simulink model "W08_0_offline"  (R2024b)
settings: Solver=ode4  StartTime=0.0  StopTime=T_end  FixedStep=Ts_ctrl  RelTol=1e-3
values from neighbouring files (symbols this model uses):
  A_Fw = 1.5    [W08_setup.m]
  A_Lw = 3.0    (= 3)    [W08_setup.m]
  alloc_mode = 2    [W08_setup.m]
  animate = 1    [W08_setup.m]
  c_n = 0.12    [W08_setup.m]
  c_x = 0.70    (= 0.7)    [W08_setup.m]
  c_y = 0.85    [W08_setup.m]
  del_max = deg2rad(45)    [W08_setup.m]
  del_rate = deg2rad(30)    [W08_setup.m]
  dp_E0 = 0    [W08_setup.m]
  dp_mode = 1    [W08_setup.m]
  dp_N0 = 0    [W08_setup.m]
  dp_PSI0 = deg2rad(0)    [W08_setup.m]
  dp_ref_on = 1    [W08_setup.m]
  dp_step = [  0    0     0    0 ... (first row only)    [W08_setup.m]
  dp_vmax = [0.5; 0.5; deg2rad(8)]    [W08_setup.m]
  F_max = 500    [W08_setup.m]
  filt_on = 1    [W08_setup.m]
  i_max = [ 200; 200; 400 ]    [W08_setup.m]
  k_wave = 900    [W08_setup.m]
  Kd_dp = diag([  110,   110,   200 ])    [W08_setup.m]
  Ki_dp = diag([    5,     5,    16 ])    [W08_setup.m]
  Kp_dp = diag([   50,    50,   160 ])    [W08_setup.m]
  L_oa = 4.9    [W08_setup.m]
  lw_arm = 1.2    [W08_setup.m]
  plant_par = [m_usv; Izz; Xu; Xuu; Yv; Yvv; Nr; Nrr]    [W08_setup.m]
  rho_air = 1.225    [W08_setup.m]
  T_e = [     1,      0,      1,      0 ... (first row only)    [W08_setup.m]
  T_pinv = pinv(T_e)    [W08_setup.m]    (also in W08_sway_demo.m = evalin('base','T_pinv'); W10_sway_demo.m = evalin('base','T_pinv'))
  tau_del = 0.20    (= 0.2)    [W08_setup.m]
  tau_n = 0.30    (= 0.3)    [W08_setup.m]
  tau_ref = 6    [W08_setup.m]
  Ts_ctrl = 0.05    [W08_setup.m]
  w_filt = 1.20    (= 1.2)    [W08_setup.m]
  wave_dir = deg2rad(45)    [W08_setup.m]
  wave_on = 1    [W08_setup.m]
  wave_par = [w_i, A_i, phi_i]    [W08_setup.m]
  wind_dir = deg2rad(45)    [W08_setup.m]
  wind_on = 1    [W08_setup.m]
  wind_speed = 6.0    (= 6)    [W08_setup.m]
  x0 = [0; 0; 0; 0; 0; 0]    [W08_setup.m]    (also in W08_vrx_run.m = x0old;   x0(6) = psi0;   assignin('base','x0', x0))
settings Model: Creator=admin  LastModifiedBy=admin

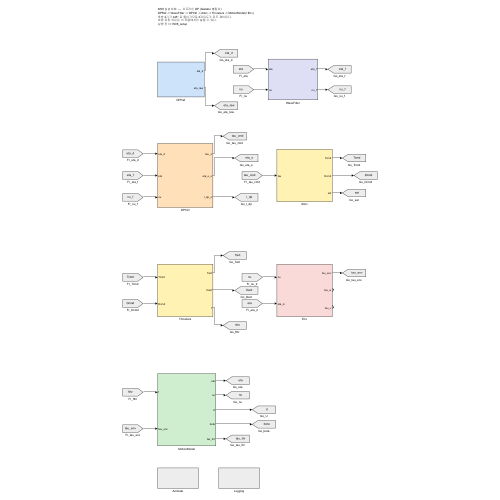
[thumbnail: Simulink's stored preview of the top-level diagram]
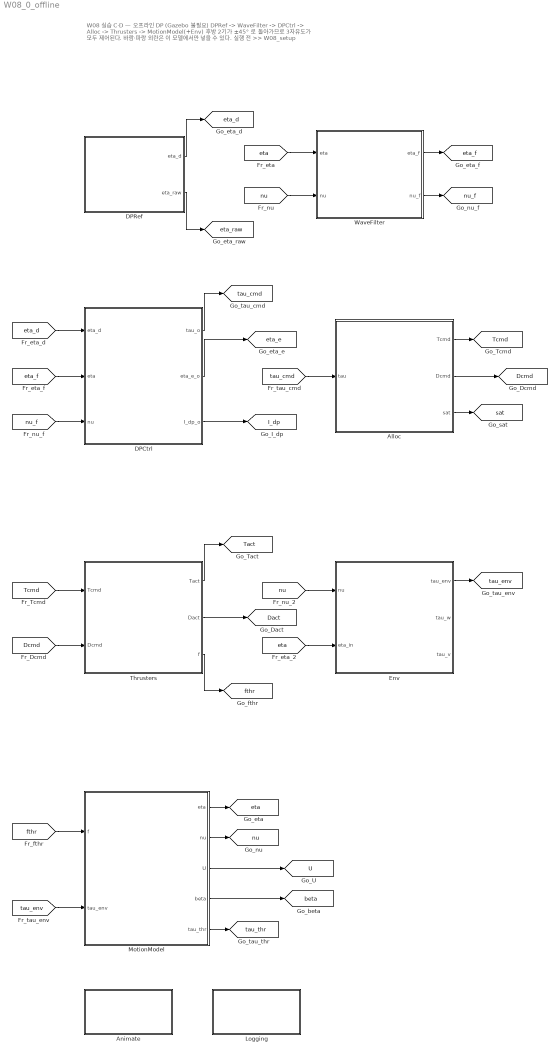
== system W08_0_offline ==
  note: W08 실습 C·D  —  오프라인 DP (Gazebo 불필요)
      | DPRef -> WaveFilter -> DPCtrl -> Alloc -> Thrusters -> MotionModel(+Env)
      | 후방 2기가 ±45° 로 돌아가므로 3자유도가 모두 제어된다.
      | 바람·파랑 외란은 이 모델에서만 넣을 수 있다.
      | 실행 전 >> W08_setup
  Alloc : Subsystem
  Animate : Subsystem
  DPCtrl : Subsystem
  DPRef : Subsystem
  Env : Subsystem
  Logging : Subsystem
  MotionModel : Subsystem
  Thrusters : Subsystem
  WaveFilter : Subsystem
  tag scope: Dact=global, Dcmd=global, I_dp=global, Tact=global, Tcmd=global, U=global, beta=global, eta=global, eta_d=global, eta_e=global, eta_f=global, eta_raw=global, fthr=global, nu=global, nu_f=global, sat=global, tau_cmd=global, tau_env=global, tau_thr=global
  wires:
  [tau_env] -> MotionModel/2(tau_env)
  [fthr] -> MotionModel/1(f)
  [eta] -> Env/2(eta_in)
  [nu] -> Env/1(nu)
  [Dcmd] -> Thrusters/2(Dcmd)
  [Tcmd] -> Thrusters/1(Tcmd)
  [tau_cmd] -> Alloc/1(tau)
  [nu_f] -> DPCtrl/3(nu)
  [eta_f] -> DPCtrl/2(eta)
  [eta_d] -> DPCtrl/1(eta_d)
  [nu] -> WaveFilter/2(nu)
  [eta] -> WaveFilter/1(eta)
  Thrusters/2(Dact) -> [Dact]
  Alloc/2(Dcmd) -> [Dcmd]
  DPCtrl/3(I_dp_o) -> [I_dp]
  Thrusters/1(Tact) -> [Tact]
  Alloc/1(Tcmd) -> [Tcmd]
  MotionModel/3(U) -> [U]
  MotionModel/4(beta) -> [beta]
  MotionModel/1(eta) -> [eta]
  DPRef/1(eta_d) -> [eta_d]
  DPCtrl/2(eta_e_o) -> [eta_e]
  WaveFilter/1(eta_f) -> [eta_f]
  DPRef/2(eta_raw) -> [eta_raw]
  Thrusters/3(f) -> [fthr]
  MotionModel/2(nu) -> [nu]
  WaveFilter/2(nu_f) -> [nu_f]
  Alloc/3(sat) -> [sat]
  DPCtrl/1(tau_o) -> [tau_cmd]
  Env/1(tau_env) -> [tau_env]
  MotionModel/5(tau_thr) -> [tau_thr]

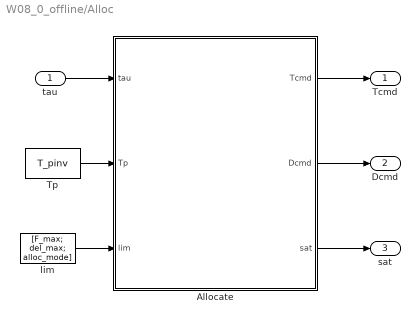
== system W08_0_offline/Alloc ==
  tau : Inport
  Allocate : MATLAB Function  TreatAsAtomicUnit=on
  Tp : Constant  Value=T_pinv
  lim : Constant  Value=[F_max; del_max; alloc_mode]
  Tcmd : Outport
  Dcmd : Outport  Port=2
  sat : Outport  Port=3
  wires:
  lim/1 -> Allocate/3(lim)
  tau/1 -> Allocate/1(tau)
  Allocate/2(Dcmd) -> Dcmd/1
  Tp/1 -> Allocate/2(Tp)
  Allocate/1(Tcmd) -> Tcmd/1
  Allocate/3(sat) -> sat/1

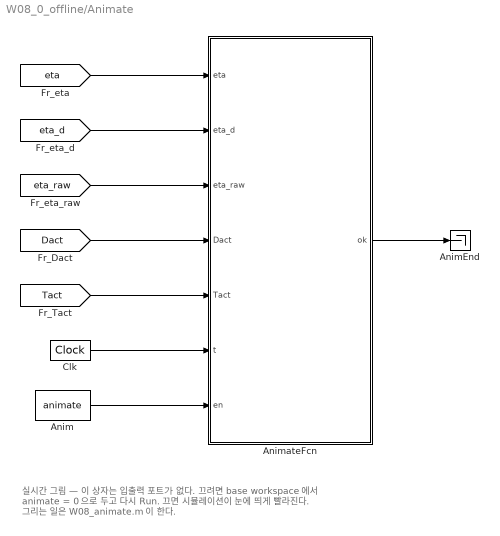
== system W08_0_offline/Animate ==
  note: 실시간 그림 — 이 상자는 입출력 포트가 없다.
      | 끄려면 base workspace 에서  animate = 0  으로 두고 다시 Run.
      | 끄면 시뮬레이션이 눈에 띄게 빨라진다.
      | 그리는 일은 W08_animate.m 이 한다.
  Anim : Constant  Value=animate
  AnimEnd : Terminator
  AnimateFcn : MATLAB Function  TreatAsAtomicUnit=on
  Clk : DigitalClock  SampleTime=Ts_ctrl
  wires:
  [eta] -> AnimateFcn/1(eta)
  [eta_d] -> AnimateFcn/2(eta_d)
  [eta_raw] -> AnimateFcn/3(eta_raw)
  [Dact] -> AnimateFcn/4(Dact)
  [Tact] -> AnimateFcn/5(Tact)
  Clk/1 -> AnimateFcn/6(t)
  Anim/1 -> AnimateFcn/7(en)
  AnimateFcn/1(ok) -> AnimEnd/1

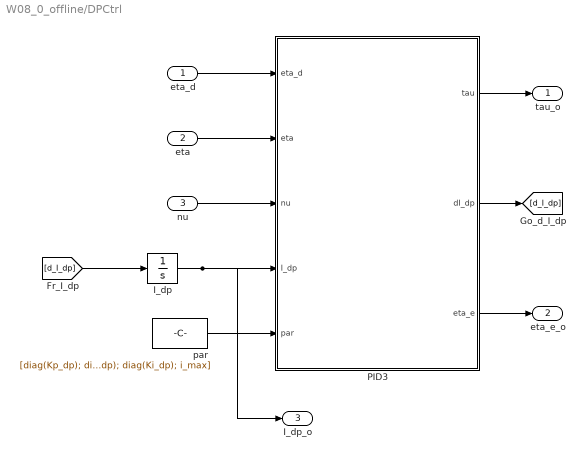
== system W08_0_offline/DPCtrl ==
  eta_d : Inport
  eta : Inport  Port=2
  nu : Inport  Port=3
  I_dp : Integrator  InitialCondition=[0;0;0]
  PID3 : MATLAB Function  TreatAsAtomicUnit=on
  par : Constant  Value=[diag(Kp_dp); diag(Kd_dp); diag(Ki_dp); i_max]
  tau_o : Outport
  eta_e_o : Outport  Port=2
  I_dp_o : Outport  Port=3
  wires:
  [d_I_dp] -> I_dp/1
  I_dp/1 -> PID3/4(I_dp), I_dp_o/1
  eta_d/1 -> PID3/1(eta_d)
  PID3/1(tau) -> tau_o/1
  eta/1 -> PID3/2(eta)
  par/1 -> PID3/5(par)
  nu/1 -> PID3/3(nu)
  PID3/2(dI_dp) -> [d_I_dp]
  PID3/3(eta_e) -> eta_e_o/1

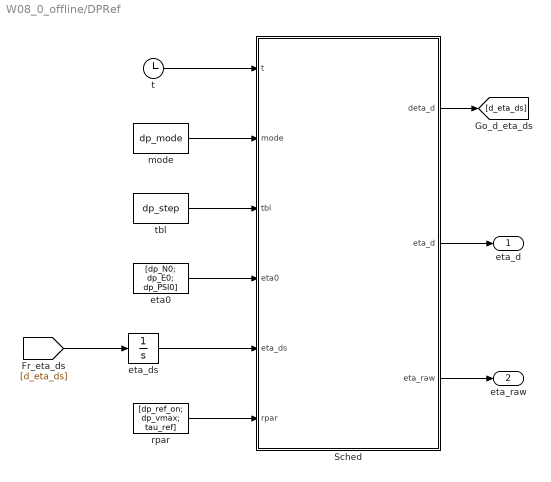
== system W08_0_offline/DPRef ==
  Sched : MATLAB Function  TreatAsAtomicUnit=on
  eta0 : Constant  Value=[dp_N0; dp_E0; dp_PSI0]
  eta_ds : Integrator  InitialCondition=[dp_N0; dp_E0; dp_PSI0]
  mode : Constant  Value=dp_mode
  rpar : Constant  Value=[dp_ref_on; dp_vmax; tau_ref]
  t : Clock
  tbl : Constant  Value=dp_step
  eta_d : Outport
  eta_raw : Outport  Port=2
  wires:
  [d_eta_ds] -> eta_ds/1
  Sched/1(deta_d) -> [d_eta_ds]
  t/1 -> Sched/1(t)
  mode/1 -> Sched/2(mode)
  eta_ds/1 -> Sched/5(eta_ds)
  tbl/1 -> Sched/3(tbl)
  eta0/1 -> Sched/4(eta0)
  rpar/1 -> Sched/6(rpar)
  Sched/2(eta_d) -> eta_d/1
  Sched/3(eta_raw) -> eta_raw/1

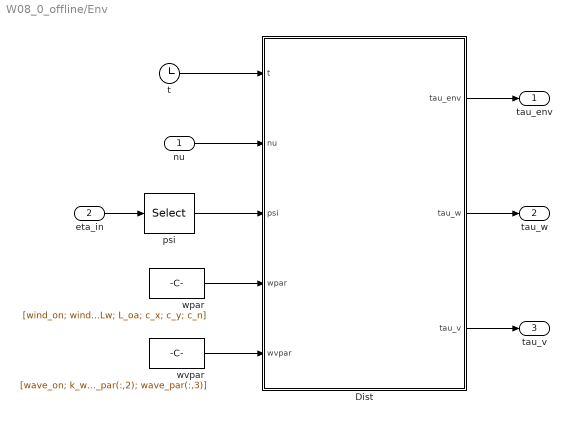
== system W08_0_offline/Env ==
  nu : Inport
  eta_in : Inport  Port=2
  Dist : MATLAB Function  TreatAsAtomicUnit=on
  psi : Selector  InputPortWidth=3  IndexOptions=Index vector (dialog)  Indices=3  OutputSizes=1
  t : Clock
  wpar : Constant  Value=[wind_on; wind_speed; wind_dir; rho_air; A_Fw; A_Lw; L_oa; c_x; c_y; c_n]
  wvpar : Constant  Value=[wave_on; k_wave; wave_dir; lw_arm; wave_par(:,1); wave_par(:,2); wave_par(:,3)]
  tau_env : Outport
  tau_w : Outport  Port=2
  tau_v : Outport  Port=3
  wires:
  eta_in/1 -> psi/1
  Dist/1(tau_env) -> tau_env/1
  t/1 -> Dist/1(t)
  nu/1 -> Dist/2(nu)
  psi/1 -> Dist/3(psi)
  wvpar/1 -> Dist/5(wvpar)
  Dist/3(tau_v) -> tau_v/1
  wpar/1 -> Dist/4(wpar)
  Dist/2(tau_w) -> tau_w/1

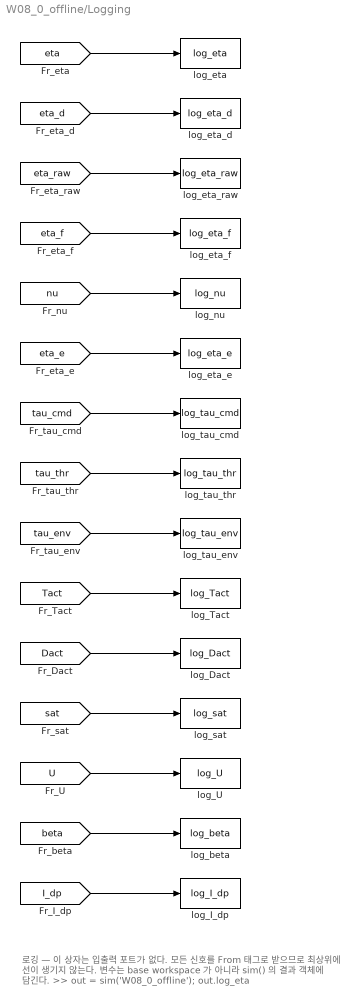
== system W08_0_offline/Logging ==
  note: 로깅 — 이 상자는 입출력 포트가 없다.
      | 모든 신호를 From 태그로 받으므로 최상위에 선이 생기지 않는다.
      | 변수는 base workspace 가 아니라 sim() 의 결과 객체에 담긴다.
      |   >> out = sim('W08_0_offline');  out.log_eta
  log_Dact : ToWorkspace  VariableName=log_Dact  SaveFormat=Timeseries  SampleTime=Ts_ctrl
  log_I_dp : ToWorkspace  VariableName=log_I_dp  SaveFormat=Timeseries  SampleTime=Ts_ctrl
  log_Tact : ToWorkspace  VariableName=log_Tact  SaveFormat=Timeseries  SampleTime=Ts_ctrl
  log_U : ToWorkspace  VariableName=log_U  SaveFormat=Timeseries  SampleTime=Ts_ctrl
  log_beta : ToWorkspace  VariableName=log_beta  SaveFormat=Timeseries  SampleTime=Ts_ctrl
  log_eta : ToWorkspace  VariableName=log_eta  SaveFormat=Timeseries  SampleTime=Ts_ctrl
  log_eta_d : ToWorkspace  VariableName=log_eta_d  SaveFormat=Timeseries  SampleTime=Ts_ctrl
  log_eta_e : ToWorkspace  VariableName=log_eta_e  SaveFormat=Timeseries  SampleTime=Ts_ctrl
  log_eta_f : ToWorkspace  VariableName=log_eta_f  SaveFormat=Timeseries  SampleTime=Ts_ctrl
  log_eta_raw : ToWorkspace  VariableName=log_eta_raw  SaveFormat=Timeseries  SampleTime=Ts_ctrl
  log_nu : ToWorkspace  VariableName=log_nu  SaveFormat=Timeseries  SampleTime=Ts_ctrl
  log_sat : ToWorkspace  VariableName=log_sat  SaveFormat=Timeseries  SampleTime=Ts_ctrl
  log_tau_cmd : ToWorkspace  VariableName=log_tau_cmd  SaveFormat=Timeseries  SampleTime=Ts_ctrl
  log_tau_env : ToWorkspace  VariableName=log_tau_env  SaveFormat=Timeseries  SampleTime=Ts_ctrl
  log_tau_thr : ToWorkspace  VariableName=log_tau_thr  SaveFormat=Timeseries  SampleTime=Ts_ctrl
  wires:
  [eta] -> log_eta/1
  [eta_d] -> log_eta_d/1
  [eta_raw] -> log_eta_raw/1
  [eta_f] -> log_eta_f/1
  [nu] -> log_nu/1
  [eta_e] -> log_eta_e/1
  [tau_cmd] -> log_tau_cmd/1
  [tau_thr] -> log_tau_thr/1
  [tau_env] -> log_tau_env/1
  [Tact] -> log_Tact/1
  [Dact] -> log_Dact/1
  [sat] -> log_sat/1
  [U] -> log_U/1
  [beta] -> log_beta/1
  [I_dp] -> log_I_dp/1

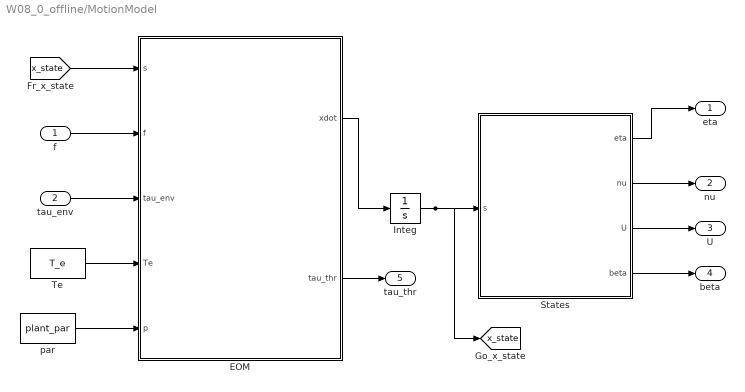
== system W08_0_offline/MotionModel ==
  f : Inport
  tau_env : Inport  Port=2
  EOM : MATLAB Function  TreatAsAtomicUnit=on
  Integ : Integrator  InitialCondition=x0
  States : MATLAB Function  TreatAsAtomicUnit=on
  Te : Constant  Value=T_e
  par : Constant  Value=plant_par
  eta : Outport
  nu : Outport  Port=2
  U : Outport  Port=3
  beta : Outport  Port=4
  tau_thr : Outport  Port=5
  tag scope: x_state=global
  wires:
  f/1 -> EOM/2(f)
  [x_state] -> EOM/1(s)
  EOM/1(xdot) -> Integ/1
  tau_env/1 -> EOM/3(tau_env)
  par/1 -> EOM/5(p)
  Te/1 -> EOM/4(Te)
  Integ/1 -> States/1(s), [x_state]
  EOM/2(tau_thr) -> tau_thr/1
  States/1(eta) -> eta/1
  States/2(nu) -> nu/1
  States/3(U) -> U/1
  States/4(beta) -> beta/1

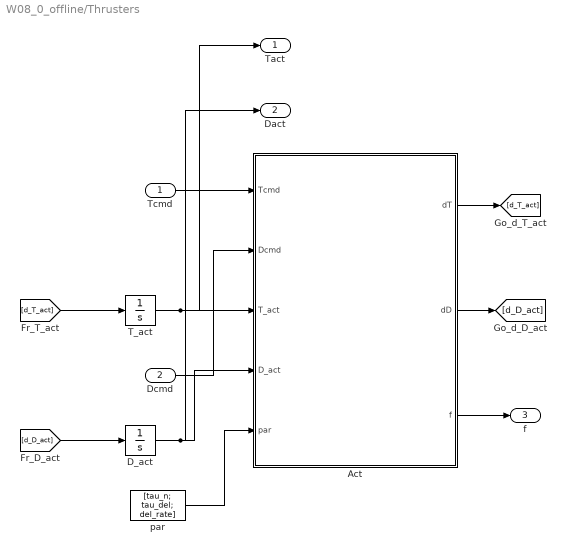
== system W08_0_offline/Thrusters ==
  Tcmd : Inport
  Dcmd : Inport  Port=2
  Act : MATLAB Function  TreatAsAtomicUnit=on
  D_act : Integrator  InitialCondition=[0;0]
  T_act : Integrator  InitialCondition=[0;0]
  par : Constant  Value=[tau_n; tau_del; del_rate]
  Tact : Outport
  Dact : Outport  Port=2
  f : Outport  Port=3
  wires:
  [d_T_act] -> T_act/1
  Tcmd/1 -> Act/1(Tcmd)
  [d_D_act] -> D_act/1
  T_act/1 -> Tact/1, Act/3(T_act)
  Act/1(dT) -> [d_T_act]
  par/1 -> Act/5(par)
  Dcmd/1 -> Act/2(Dcmd)
  D_act/1 -> Dact/1, Act/4(D_act)
  Act/2(dD) -> [d_D_act]
  Act/3(f) -> f/1

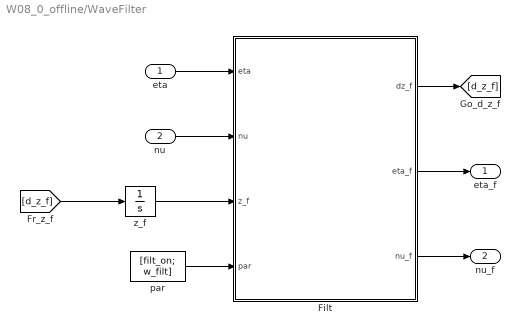
== system W08_0_offline/WaveFilter ==
  eta : Inport
  nu : Inport  Port=2
  Filt : MATLAB Function  TreatAsAtomicUnit=on
  par : Constant  Value=[filt_on; w_filt]
  z_f : Integrator  InitialCondition=[0;0;0;0;0;0]
  eta_f : Outport
  nu_f : Outport  Port=2
  wires:
  [d_z_f] -> z_f/1
  Filt/2(eta_f) -> eta_f/1
  par/1 -> Filt/4(par)
  z_f/1 -> Filt/3(z_f)
  eta/1 -> Filt/1(eta)
  nu/1 -> Filt/2(nu)
  Filt/1(dz_f) -> [d_z_f]
  Filt/3(nu_f) -> nu_f/1

== matlab function W08_0_offline/MotionModel/States ==
  data: s input; eta output; nu output; U output; beta output
function [eta, nu, U, beta] = States(s)
%#codegen
nu   = s(1:3);
eta  = s(4:6);
U    = sqrt(s(1)*s(1) + s(2)*s(2));
beta = atan2(s(2), s(1));

== matlab function W08_0_offline/Animate/AnimateFcn ==
  data: eta input; ok output; eta_d input; eta_raw input; Dact input; Tact input; t input; en input
function ok = AnimateFcn(eta, eta_d, eta_raw, Dact, Tact, t, en)
%#codegen
% Live plot while the model runs. A MATLAB Function block cannot
% plot, so the drawing function is declared extrinsic: Simulink
% calls plain MATLAB instead of generating code for it.
coder.extrinsic('W08_animate');
ok = 1;
if en > 0.5
    W08_animate(eta, eta_d, eta_raw, Dact, Tact, t);
end

== matlab function W08_0_offline/WaveFilter/Filt ==
  data: eta input; dz_f output; nu input; z_f input; par input; eta_f output; nu_f output
function [dz_f, eta_f, nu_f] = Filt(eta, nu, z_f, par)
%#codegen
% Wave filtering for dynamic positioning.
%
% First order wave loads make the vessel oscillate at the wave
% frequency. That motion cannot be counteracted — trying to do so
% only wears out the thrusters. A DP system therefore feeds the
% controller with the LOW FREQUENCY part of the motion only.
% Fossen (2011) 11.4.1 uses a passive observer; here a first order
% low pass with a cut-off well below the wave frequency is enough to
% show the effect.
%
% CONTINUOUS TIME:   dz_f/dt = wf * (z - z_f)
% An Integrator holds z_f, so the cut-off wf is the only number here.
%
% par = [on; wf]

on = par(1); wf = par(2);
z  = [eta; nu];
dz_f = zeros(6,1);
if on < 0.5
    eta_f = eta;  nu_f = nu;
    return
end
d = z - z_f;
% heading must be filtered on the difference, not the raw angle
d(3) = atan2(sin(d(3)), cos(d(3)));
dz_f = wf * d;
eta_f = z_f(1:3);
nu_f  = z_f(4:6);

== matlab function W08_0_offline/DPRef/Sched ==
  data: t input; deta_d output; mode input; tbl input; eta0 input; eta_ds input; rpar input; eta_d output; eta_raw output
function [deta_d, eta_d, eta_raw] = Sched(t, mode, tbl, eta0, eta_ds, rpar)
%#codegen
% DP setpoint scheduler and REFERENCE MODEL.
%
%   mode 0 : hold the initial setpoint
%   mode 1 : step through the table  [t  N  E  psi_deg]
%
% A raw step demand is never given to a DP controller. The vessel
% cannot move at any speed, so a step makes the controller ask for a
% force the thrusters cannot deliver, and the loop saturates.
% A reference model turns the step into a feasible trajectory. Here a
% saturated proportional law is used:
%     v = (eta_raw - eta_d)/tau_ref,   |v| <= v_max
% Far from the target the setpoint moves at the constant speed v_max;
% close to it the approach becomes exponential with time constant
% tau_ref, so there is no corner at arrival.
% Fossen (2011) calls this the reference model; every DP system has
% one.
%
% CONTINUOUS TIME. The function returns the RATE of the setpoint and
% an Integrator holds the state, so the law above is written exactly
% as it stands - no Ts anywhere.
%
% rpar = [on; vx; vy; vPsi; tau_ref]

eta_raw = eta0;
if mode > 0.5
    n = size(tbl,1);
    for i = 1:n
        if t >= tbl(i,1)
            eta_raw = [tbl(i,2); tbl(i,3); tbl(i,4)*pi/180];
        end
    end
end

deta_d = zeros(3,1);
if rpar(1) < 0.5
    eta_d = eta_raw;        % reference model off: the step goes straight through
    return
end

vmax = rpar(2:4);  tr = rpar(5);
for i = 1:3
    d = eta_raw(i) - eta_ds(i);
    if i == 3, d = atan2(sin(d), cos(d)); end
    v = d/tr;
    if v >  vmax(i), v =  vmax(i); end
    if v < -vmax(i), v = -vmax(i); end
    deta_d(i) = v;
end
eta_d = eta_ds;

== matlab function W08_0_offline/DPCtrl/PID3 ==
  data: eta_d input; tau output; eta input; nu input; I_dp input; par input; dI_dp output; eta_e output
function [tau, dI_dp, eta_e] = PID3(eta_d, eta, nu, I_dp, par)
%#codegen
% 3-DOF dynamic positioning controller (Fossen 2011, 12.2.10).
%
%   eta   = [N; E; psi]      position and heading in NED
%   nu    = [u; v; r]        velocity in BODY
%   tau   = -J(psi)' * (Kp*eta_e + Ki*I) - Kd*nu
%
% The transpose of the rotation matrix turns a NED position error into
% a BODY force. Damping is taken on BODY velocity directly, so no
% derivative of the error is needed (same idea as the P-D heading
% controller of week 7).
%
% CONTINUOUS TIME. The function returns dI/dt = e and an Integrator
% holds I, so the integral term is a true 1/s - there is no Ts here.
%
% par = [Kp(1:3); Kd(1:3); Ki(1:3); imax(1:3)]

Kp = par(1:3);  Kd = par(4:6);  Ki = par(7:9);  im = par(10:12);

e = eta - eta_d;
e(3) = atan2(sin(e(3)), cos(e(3)));      % smallest signed angle

psi = eta(3);
J = [ cos(psi), -sin(psi), 0;
      sin(psi),  cos(psi), 0;
             0,         0, 1];

% CLAMPING anti-windup: at the limit, and still being pushed further
% out, the integral simply stops. Same rule the PI blocks of weeks
% 4-7 use, written out because the law here is 3-DOF.
dI_dp = e;
for i = 1:3
    lim = im(i)/max(Ki(i), 1e-9);
    if (I_dp(i) >=  lim && e(i) > 0) || (I_dp(i) <= -lim && e(i) < 0)
        dI_dp(i) = 0;
    end
end

tau = -J' * ( Kp.*e + Ki.*I_dp ) - Kd.*nu;
eta_e = e;

== matlab function W08_0_offline/Alloc/Allocate ==
  data: tau input; Tcmd output; Tp input; lim input; Dcmd output; sat output
function [Tcmd, Dcmd, sat] = Allocate(tau, Tp, lim)
%#codegen
% Thrust allocation for two azimuth (rotatable) thrusters.
% Fossen (2011) 12.3.4 — constrained control allocation for azimuth
% thrusters, solved with the EXTENDED THRUST VECTOR.
%
% Step 1  f = pinv(T_e) * tau       f = [FxL FyL FxR FyR]'
%         Because the thruster force is written in Cartesian components,
%         T_e is CONSTANT and its pseudo-inverse can be precomputed.
%         There is no singular configuration to worry about.
%
% Step 2  Cartesian -> polar   T = |f_i|,  delta = atan2(Fy, Fx)
%
% Step 3  map the demand into the mechanical sector |delta| <= 45 deg
%           |d| <=  45  : use as is
%           |d| >  135  : REVERSE thrust, d -> d -+ 180
%           otherwise   : dead zone, no thrust can be produced
%
% Step 4  saturate the magnitude at F_max
%
% lim = [F_max; delta_max; mode]
%   mode 1 : dead zone   — demands inside the forbidden sector are
%            dropped. Simple, but the realised tau is then wrong.
%   mode 2 : clamp       — the angle is pushed to the nearest sector
%            edge and the magnitude is scaled by cos of the angle
%            error, so the useful component is kept.

f = Tp * tau;
Fmax = lim(1);  dmax = lim(2);  mode = lim(3);

Tcmd = zeros(2,1);  Dcmd = zeros(2,1);  sat = 0;
for i = 1:2
    fx = f(2*i-1);  fy = f(2*i);
    Ti = sqrt(fx*fx + fy*fy);
    di = atan2(fy, fx);
    ad = abs(di);
    if ad <= dmax
        To = Ti;   Do = di;
    elseif ad >= pi - dmax
        To = -Ti;  Do = di - sign(di)*pi;    % reverse thrust
    elseif mode < 1.5
        To = 0;    Do = 0;                   % dead zone
        sat = sat + 1;
    else
        % clamp to the nearest edge of the reachable sector
        if ad <= pi/2
            Do = sign(di)*dmax;      To =  Ti*cos(ad - dmax);
        else
            Do = -sign(di)*dmax;        To = -Ti*cos(pi - dmax - ad);
            Do = atan2(sin(Do), cos(Do));
        end
        sat = sat + 1;
    end
    if To >  Fmax, To =  Fmax; sat = sat + 1; end
    if To < -Fmax, To = -Fmax; sat = sat + 1; end
    Tcmd(i) = To;  Dcmd(i) = Do;
end

== matlab function W08_0_offline/Thrusters/Act ==
  data: Tcmd input; dT output; Dcmd input; T_act input; D_act input; par input; dD output; f output
function [dT, dD, f] = Act(Tcmd, Dcmd, T_act, D_act, par)
%#codegen
% Actuator dynamics of an azimuth thruster.
%   thrust  : first order lag, time constant tau_n
%   azimuth : first order lag (tau_del) whose angular RATE is capped
%             at rate_max. A real pod cannot snap to a new angle.
%
% CONTINUOUS TIME. The function returns the two RATES and Integrators
% hold the states, so the rate cap is written on the rate itself -
% rad/s, not rad per sample.
%
%   dT/dt = (Tcmd - T)/tau_n
%   dD/dt = sat( ssa(Dcmd - D)/tau_del , +-rate_max )
%
% par = [tau_n; tau_del; rate_max]

tn = par(1); td = par(2); rmax = par(3);

dT = (Tcmd - T_act)/tn;

dD = zeros(2,1);
for i = 1:2
    dd = Dcmd(i) - D_act(i);
    dd = atan2(sin(dd), cos(dd));           % shortest way round
    rate = dd/td;                           % first order lag ...
    if rate >  rmax, rate =  rmax; end      % ... whose RATE is capped
    if rate < -rmax, rate = -rmax; end
    dD(i) = rate;
end

% back to Cartesian components in BODY
f = [ T_act(1)*cos(D_act(1));
      T_act(1)*sin(D_act(1));
      T_act(2)*cos(D_act(2));
      T_act(2)*sin(D_act(2)) ];

== matlab function W08_0_offline/Env/Dist ==
  data: t input; tau_env output; nu input; psi input; wpar input; wvpar input; tau_w output; tau_v output
function [tau_env, tau_w, tau_v] = Dist(t, nu, psi, wpar, wvpar)
%#codegen
% Environmental loads in BODY axes.
%
% WIND  — Jin et al. (2025) Eq. (11)-(19); Fossen (2011) 8.1
%   relative wind in BODY :
%     u_rw = u + Vw cos(beta_w - psi)   beta_w = direction wind COMES FROM
%     v_rw = v + Vw sin(beta_w - psi)   (Fossen uses going-to, hence minus)
%   q     = 0.5 rho_a Vrw^2
%   tau_w = q * [ CX*AFw ; CY*ALw ; CN*ALw*L ]
%   CX = -cx cos(g), CY = +cy sin(g), CN = cn sin(2g)   (Fossen 8.21)
%
% WAVE  — first order approximation. Component amplitudes come from a
%   Bretschneider spectrum (Jin et al. Eq. (21)-(25)); the force is
%   taken proportional to the surface elevation with a single gain.
%   This is an approximation, not a diffraction calculation.
%
% wpar  = [on; Vw; beta_w; rho_a; AFw; ALw; L; cx; cy; cn]
% wvpar = [on; k_wave; theta_m; arm; w1..wn; A1..An; p1..x_n]

u = nu(1); v = nu(2);
tau_w = zeros(3,1);
if wpar(1) > 0.5
    Vw = wpar(2); bw = wpar(3); rho = wpar(4);
    AF = wpar(5); AL = wpar(6); L = wpar(7);
    cx = wpar(8); cy = wpar(9); cn = wpar(10);
    urw = u + Vw*cos(bw - psi);
    vrw = v + Vw*sin(bw - psi);
    Vrw = sqrt(urw*urw + vrw*vrw);
    g   = -atan2(vrw, urw);
    q   = 0.5*rho*Vrw*Vrw;
    tau_w = q * [ -cx*cos(g)*AF;
                   cy*sin(g)*AL;
                   cn*sin(2*g)*AL*L ];
end

tau_v = zeros(3,1);
if wvpar(1) > 0.5
    kw = wvpar(2); th = wvpar(3); arm = wvpar(4);
    n  = (numel(wvpar) - 4)/3;
    zeta = 0;
    for i = 1:n
        wi = wvpar(4+i);
        Ai = wvpar(4+n+i);
        pi_i = wvpar(4+2*n+i);
        zeta = zeta + Ai*sin(wi*t + pi_i);
    end
    rel = th - psi;                          % wave direction in BODY
    Fw  = kw*zeta;
    tau_v = [ Fw*cos(rel); Fw*sin(rel); arm*Fw*sin(rel) ];
end

tau_env = tau_w + tau_v;

== matlab function W08_0_offline/MotionModel/EOM ==
  data: s input; xdot output; f input; tau_env input; Te input; p input; tau_thr output
function [xdot, tau_thr] = EOM(s, f, tau_env, Te, p)
%#codegen
% 3-DOF WAM-V equations of motion, NED — same coefficients as weeks
% 7 to 9 (taken from the Gazebo VRX plugins).
% The only change is the input: the thruster force now has a sway
% component, so all three degrees of freedom are actuated.
%   s = [u v r N E psi]'
%   p = [m Izz Xu Xuu Yv Yvv Nr Nrr]'

u = s(1); v = s(2); r = s(3); psi = s(6);
mm=p(1); Izz=p(2); Xu=p(3); Xuu=p(4); Yv=p(5); Yvv=p(6);
Nr=p(7); Nrr=p(8);

tau_thr = Te*f;                 % [X; Y; N] from the thrusters
tau     = tau_thr + tau_env;

Dx = (Xu + Xuu*abs(u))*u;
Dy = (Yv + Yvv*abs(v))*v;
Dn = (Nr + Nrr*abs(r))*r;

du = (tau(1) - Dx)/mm + v*r;    % rigid-body Coriolis
dv = (tau(2) - Dy)/mm - u*r;
dr = (tau(3) - Dn)/Izz;

xdot = [du; dv; dr;
        u*cos(psi) - v*sin(psi);
        u*sin(psi) + v*cos(psi);
        r];
